simulink model "task1"  (R2024a)
settings: Solver=VariableStepAuto  StartTime=0.0  StopTime=10.0  MaxStep=0.01  RelTol=1e-3
values from neighbouring files (symbols this model uses):
  Init_finished = 1    [firstTask.m]
  j123_q_meas = [0.2 0.4 0.8]    [firstTask.m]
  j3_q_desired = 0.5    [firstTask.m]
settings Model: Creator=arsik  LastModifiedBy=arsik

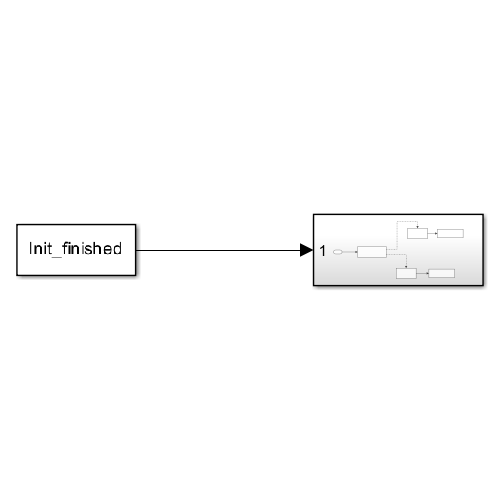
[thumbnail: Simulink's stored preview of the top-level diagram]
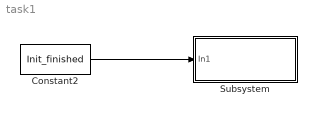
== system task1 ==
  Constant2 : Constant  Value=Init_finished
  Subsystem : Subsystem
  wires:
  Constant2/1 -> Subsystem/1(In1)

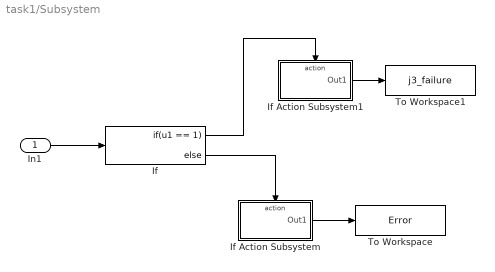
== system task1/Subsystem ==
  In1 : Inport
  If : If  IfExpression=u1 == 1
  If Action Subsystem : Subsystem  TreatAsAtomicUnit=on
  If Action Subsystem1 : Subsystem  TreatAsAtomicUnit=on
  To Workspace : ToWorkspace  VariableName=Error  SampleTime=-1
  To Workspace1 : ToWorkspace  VariableName=j3_failure  SampleTime=-1
  wires:
  In1/1 -> If/1
  If/2 -> If Action Subsystem/Action
  If/1 -> If Action Subsystem1/Action
  If Action Subsystem/1(Out1) -> To Workspace/1
  If Action Subsystem1/1(Out1) -> To Workspace1/1

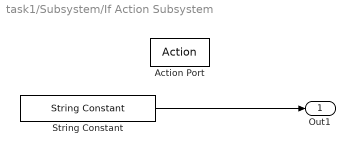
== system task1/Subsystem/If Action Subsystem ==
  Action Port : ActionPort  ActionPortLabel=else
  String Constant : StringConstant  String="\"Initialization is not finished\""
  Out1 : Outport
  wires:
  String Constant/1 -> Out1/1

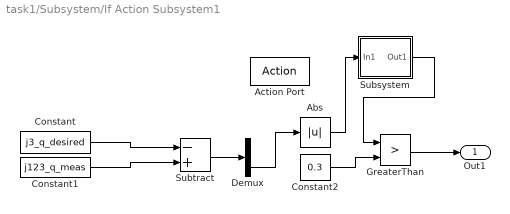
== system task1/Subsystem/If Action Subsystem1 ==
  Action Port : ActionPort  ActionPortLabel=if(u1 == 1)
  Abs : Abs  SaturateOnIntegerOverflow=off
  Constant : Constant  Value=j3_q_desired
  Constant1 : Constant  Value=j123_q_meas
  Constant2 : Constant  Value=0.3
  Demux : Demux  Outputs=3
  GreaterThan : RelationalOperator  Operator=>  OutDataTypeStr=boolean  RndMeth=Simplest  InputSameDT=off
  Subsystem : Subsystem
  Subtract : Sum  Inputs=-+
  Out1 : Outport
  wires:
  Constant1/1 -> Subtract/2
  GreaterThan/1 -> Out1/1
  Demux/3 -> Abs/1
  Constant/1 -> Subtract/1
  Constant2/1 -> GreaterThan/2
  Subtract/1 -> Demux/1
  Abs/1 -> Subsystem/1(In1)
  Subsystem/1(Out1) -> GreaterThan/1

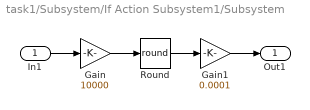
== system task1/Subsystem/If Action Subsystem1/Subsystem ==
  In1 : Inport
  Gain : Gain  Gain=10000
  Gain1 : Gain  Gain=0.0001
  Round : Rounding  Operator=round
  Out1 : Outport
  wires:
  Round/1 -> Gain1/1
  Gain/1 -> Round/1
  Gain1/1 -> Out1/1
  In1/1 -> Gain/1
